simulink library "lib_parallel_comp"  (Simulink 7.4)
settings: Solver=ode45  StartTime=0.0  StopTime=10.0  RelTol=1e-3
values from neighbouring files (symbols this model uses):
  Ts = 0.05    [const_sim.m]    (also in cost_functions.m; read_cpu_times.m; read_cpu_times_serial.m)
  uoff1 = [0.304, 0.405, 1, 0]'    [const_sim.m]
  uoff2 = [0.304, -1, 0.393, 0]'    [const_sim.m]
undefined symbols (not defined in the file or in its folder): n_delay, xinit
libraries: lib_compressor x2
settings Model: Creator=chkajon  LastModifiedBy=chkajon

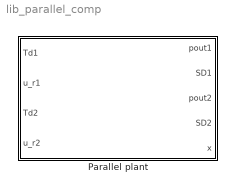
== system lib_parallel_comp ==
  Parallel plant : Subsystem  mask{x_init_total=xinit, disturbances_on=off, dist_t_in=, dist1_in=0, dist2_in=0}
      mask prompts: x_init_total "Initial state"; disturbances_on "Activate disturbances"; dist_t_in "Disturbance times (up to 2)"; dist1_in "Disturbance 1 values (u1in, u1out, u2out)"; dist2_in "Disturbance 2 values"
      mask init:
      | dist1 = zeros(3,1);
      | dist2 = dist1;
      | dist_t = zeros(2,1);
      | 
      | if disturbances_on
      |     for i=1:min(3,length(dist1_in))
      |         dist1(i) = dist1_in(i);
      |     end
      |     for i=1:min(3,length(dist2_in))
      |         dist2(i) = dist2_in(i);
      |     end
      |     for i=1:min(2,length(dist_t_in))
      |         dist_t(i) = dist_t_in(i);
      |     end
      | end
      | 
      | x_init1 = x_init_total(1:5);
      | x_init2 = x_init_total(6:10);

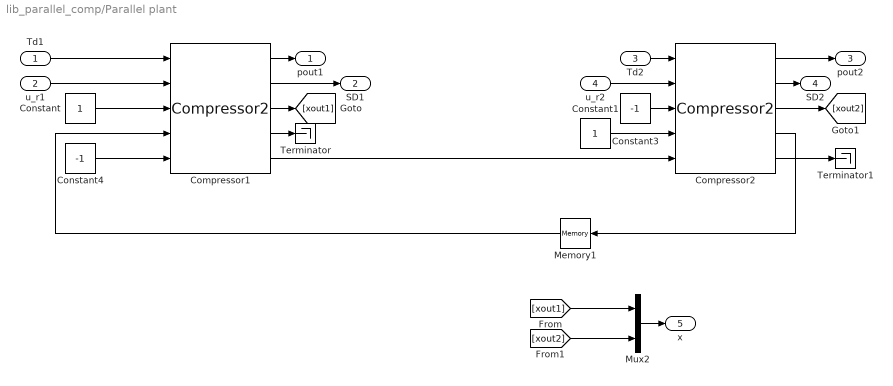
== system lib_parallel_comp/Parallel plant ==
  Td1 : Inport  OutDataType=fixdt(1, 16)  OutScaling=2^0
  u_r1 : Inport  Port=2  OutDataType=fixdt(1, 16)  OutScaling=2^0
  Td2 : Inport  Port=3  OutDataType=fixdt(1, 16)  OutScaling=2^0
  u_r2 : Inport  Port=4  OutDataType=fixdt(1, 16)  OutScaling=2^0
  Compressor1 : lib_compressor/Compressor2  SystemSampleTime=-1  x_init=x_init1  Td_off=uoff1(1)  u_in=uoff1(2)  u_out=uoff1(3)  u_rec=uoff1(4)  t_delay=n_delay(2)*Ts  use_dist=on  u_out_dist=[dist1(1); dist2(1)]  u_out_time=dist_t  u_in_dist=[dist1(2); dist2(2)]  u_in_time=dist_t
  Compressor2 : lib_compressor/Compressor2  SystemSampleTime=-1  x_init=x_init2  Td_off=uoff2(1)  u_in=uoff2(2)  u_out=uoff2(3)  u_rec=uoff2(4)  t_delay=n_delay(2)*Ts  use_dist=on  u_out_dist=[dist1(3); dist2(3)]  u_out_time=dist_t  u_in_dist=[0;0]  u_in_time=dist_t
  Constant : Constant  OutDataType=fixdt(1, 16)  OutScaling=2^0
  Constant1 : Constant  OutDataType=fixdt(1, 16)  OutScaling=2^0
  Constant3 : Constant  Value=-1  OutDataType=fixdt(1, 16)  OutScaling=2^0
  Constant4 : Constant  Value=-1  OutDataType=fixdt(1, 16)  OutScaling=2^0
  Memory1 : Memory  X0=x_init_total(6)
  Mux2 : Mux  Inputs=2
  Terminator : Terminator
  Terminator1 : Terminator
  pout1 : Outport  OutDataType=fixdt(1, 16)  OutScaling=2^0
  SD1 : Outport  Port=2  OutDataType=fixdt(1, 16)  OutScaling=2^0
  pout2 : Outport  Port=3  OutDataType=fixdt(1, 16)  OutScaling=2^0
  SD2 : Outport  Port=4  OutDataType=fixdt(1, 16)  OutScaling=2^0
  x : Outport  Port=5  OutDataType=fixdt(1, 16)  OutScaling=2^0
  wires:
  Constant4/1 -> Compressor1/5
  Constant/1 -> Compressor1/3
  u_r1/1 -> Compressor1/2
  Td1/1 -> Compressor1/1
  Compressor2/5 -> Terminator1/1
  Compressor1/4 -> Terminator/1
  Constant3/1 -> Compressor2/3
  Td2/1 -> Compressor2/1
  u_r2/1 -> Compressor2/2
  [xout1] -> Mux2/1
  [xout2] -> Mux2/2
  Mux2/1 -> x/1
  Compressor1/1 -> pout1/1
  Constant1/1 -> Compressor2/4
  Compressor1/2 -> SD1/1
  Compressor1/3 -> [xout1]
  Compressor2/1 -> pout2/1
  Compressor2/2 -> SD2/1
  Compressor2/3 -> [xout2]
  Compressor2/4 -> Memory1/1
  Memory1/1 -> Compressor1/4
  Compressor1/5 -> Compressor2/5
